simulink model "w3p2"  (R2020b)
settings: Solver=VariableStepAuto  StartTime=0.0  StopTime=10.0  RelTol=1e-3
settings Model: Creator=Dell  LastModifiedBy=Dell

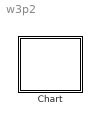
== system w3p2 ==
  Chart : Stateflow chart  TreatAsAtomicUnit=on

== stateflow chart w3p2/Chart ==
  state Stop
    en:
    y1=RED;
    y2=GREEN;
  state StopForTraffic
    en:
    y1=RED;
    y2=GREEN;
  state StopToGo
    en:
    y1=RED;
    y2=YELLOW;
  state GoToStop
    en:
    y1=YELLOW;
    y2=RED;
  state Go
    en:
    y1=GREEN;
    y2=RED;
  (default) -> Stop
  Stop -> StopForTraffic : after(20,tick)
  StopForTraffic -> StopToGo : [sens]
  GoToStop -> Stop : after(3,tick)
  StopToGo -> Go : after(3,tick)
  Go -> GoToStop : after(10,tick)
